simulink model "Buck_closed_loop"  (R2013a)
settings: Solver=ode45  StartTime=0.0  StopTime=0.003  MaxStep=0.1e-6  RelTol=1e-3
libraries: simulink x1
settings Model: Creator=Rony  LastModifiedBy=Rony

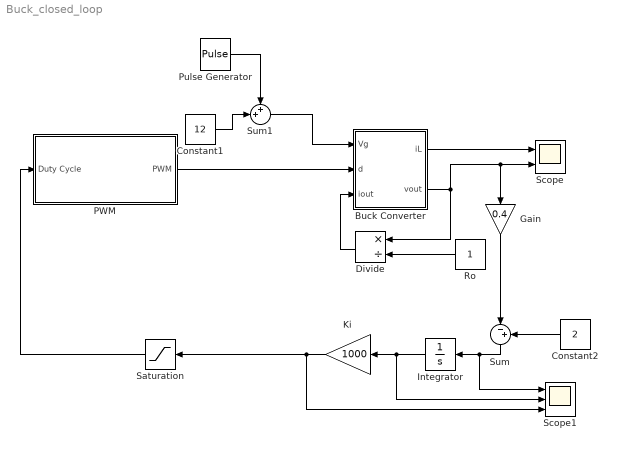
== system Buck_closed_loop ==
  Buck Converter : Subsystem
  Constant1 : Constant  Value=12
  Constant2 : Constant  Value=2
  Divide : Product  Inputs=*/
  Gain : Gain  Gain=0.4
  Integrator : Integrator  UpperSaturationLimit=0.9/1000  LowerSaturationLimit=0.1/1000
  Ki : Gain  Gain=1000
  PWM : Subsystem
  Pulse Generator : DiscretePulseGenerator  PulseType=Time based  Amplitude=6  Period=0.003  PulseWidth=50
  Ro : Constant
  Saturation : Saturate  UpperLimit=0.9  LowerLimit=0.1
  Scope : Scope  NumInputPorts=2
      settings: TimeRange=0.003  YMin=0~4.5  YMax=10~6
  Scope1 : Scope  NumInputPorts=3
      settings: YMin=0~4.9~-5  YMax=10~5.1~5
  Sum : Sum  Inputs=|-+
  Sum1 : Sum  Inputs=++|
  wires:
  Divide/1 -> Buck Converter/3(iout)
  Buck Converter/1(iL) -> Scope/1
  Buck Converter/2("vout ") -> Gain/1, Scope/2, Divide/1
  Ki/1 -> Saturation/1, Scope1/3
  PWM/1(PWM) -> Buck Converter/2(d)
  Gain/1 -> Sum/1
  Constant2/1 -> Sum/2
  Sum/1 -> Scope1/1, Integrator/1
  Integrator/1 -> Scope1/2, Ki/1
  Ro/1 -> Divide/2
  Constant1/1 -> Sum1/2
  Pulse Generator/1 -> Sum1/1
  Sum1/1 -> Buck Converter/1(Vg)
  Saturation/1 -> PWM/1(Duty Cycle)

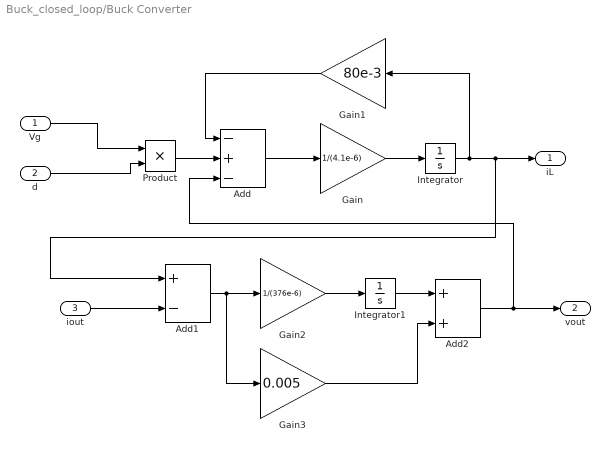
== system Buck_closed_loop/Buck Converter ==
  Vg : Inport
  d : Inport  Port=2
  iout : Inport  Port=3
  Add : Sum  Inputs=-+-
  Add1 : Sum  Inputs=+-
  Add2 : Sum
  Gain : Gain  Gain=1/(4.1e-6)
  Gain1 : Gain  Gain=80e-3
  Gain2 : Gain  Gain=1/(376e-6)
  Gain3 : Gain  Gain=0.005
  Integrator : Integrator
  Integrator1 : Integrator
  Product : Product
  iL : Outport
  "vout " : Outport  Port=2
  wires:
  Add/1 -> Gain/1
  Vg/1 -> Product/1
  d/1 -> Product/2
  Add2/1 -> "vout "/1, Add/3
  Gain/1 -> Integrator/1
  Integrator/1 -> iL/1, Add1/1, Gain1/1
  Product/1 -> Add/2
  Integrator1/1 -> Add2/1
  Add1/1 -> Gain3/1, Gain2/1
  Gain3/1 -> Add2/2
  Gain1/1 -> Add/1
  iout/1 -> Add1/2
  Gain2/1 -> Integrator1/1

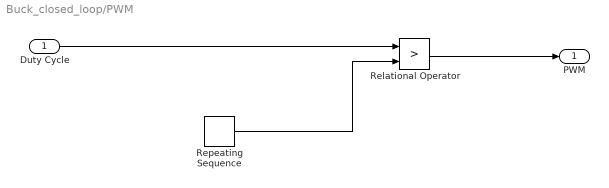
== system Buck_closed_loop/PWM ==
  Duty Cycle : Inport
  Relational Operator : RelationalOperator  Operator=>  OutDataTypeStr=boolean
  Repeating Sequence : simulink/Sources/Repeating Sequence  rep_seq_t=[0 0.001e-5 1e-5]  rep_seq_y=[1 0 1]
  PWM : Outport
  wires:
  Relational Operator/1 -> PWM/1
  Repeating Sequence/1 -> Relational Operator/2
  Duty Cycle/1 -> Relational Operator/1
